simulink model "Task2"  (R2022a)
settings: Solver=FixedStepAuto  StartTime=0.0  StopTime=10.0  FixedStep=0.0001  RelTol=1e-3
undefined symbols (not defined in the file): a_0, a_1, s1, s2
settings Model: Creator=Family  LastModifiedBy=Family

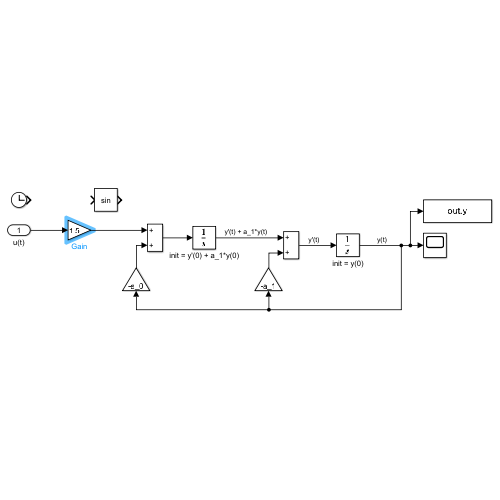
[thumbnail: Simulink's stored preview of the top-level diagram]
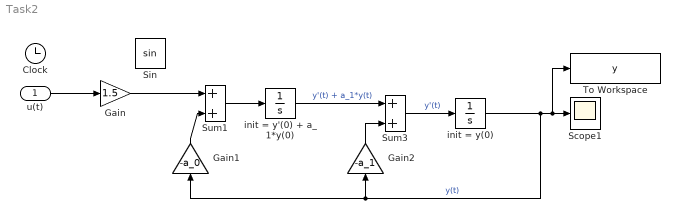
== system Task2 ==
  u(t) : Inport
  Clock : Clock
  Gain : Gain  Gain=1.5
  Gain1 : Gain  Gain=-a_0
  Gain2 : Gain  Gain=-a_1
  Scope1 : Scope
  Sin : Trigonometry
  Sum1 : Sum
  Sum3 : Sum
  To Workspace : ToWorkspace  VariableName=y  SaveFormat=Timeseries  SampleTime=-1
  init = y'(0) + a_1*y(0) : Integrator  InitialCondition=s2
  init = y(0) : Integrator  InitialCondition=s1
  wires:
  Sum1/1 -> init = y'(0) + a_1*y(0)/1
  Gain1/1 -> Sum1/2
  init = y'(0) + a_1*y(0)/1 -> Sum3/1  "y'(t) + a_1*y(t)"
  Gain2/1 -> Sum3/2
  init = y(0)/1 -> To Workspace/1, Scope1/1, Gain1/1, Gain2/1  "y(t)"
  Sum3/1 -> init = y(0)/1  "y'(t)"
  Gain/1 -> Sum1/1
  u(t)/1 -> Gain/1
